simulink model "my_dom_trans_2013"  (R2013a)
settings: Solver=ode45  SolverMode=SingleTasking  StartTime=0.0  StopTime=10000  RelTol=1e-3
undefined symbols (not defined in the file): d_T_z, d_T_zew, L1, L2, M1, M2, steptime, T_p0, T_wew0
settings Model: CovMetricSettings=dwe  CovHtmlReporting=off  covSaveCumulativeToWorkspaceVar=off  CovSaveSingleToWorkspaceVar=off  CovExternalEMLEnable=on  Creator=johnb  LastModifiedBy=johnb
settings DataIOCC: LimitDataPoints=off  SaveFormat=StructureWithTime
settings DebuggingCC: UnderspecifiedInitializationDetection=Simplified  MergeDetectMultiDrivingBlocksExec=error  SolverPrmCheckMsg=none  FrameProcessingCompatibilityMsg=error  StateNameClashWarn=none  SFUnexpectedBacktrackingDiag=error  SFNoUnconditionalDefaultTransitionDiag=error
settings HardwareCC: ProdBitPerPointer=64  ProdLargestAtomicFloat=Float  ProdIntDivRoundTo=Zero  ProdEndianess=LittleEndian  ProdHWDeviceType=Specified
settings ModelReferenceCC: PropagateSignalLabelsOutOfModel=on
settings GRTTargetCC: CodeReplacementLibrary=C99 (ISO)  GeneratePreprocessorConditionals=Use local settings

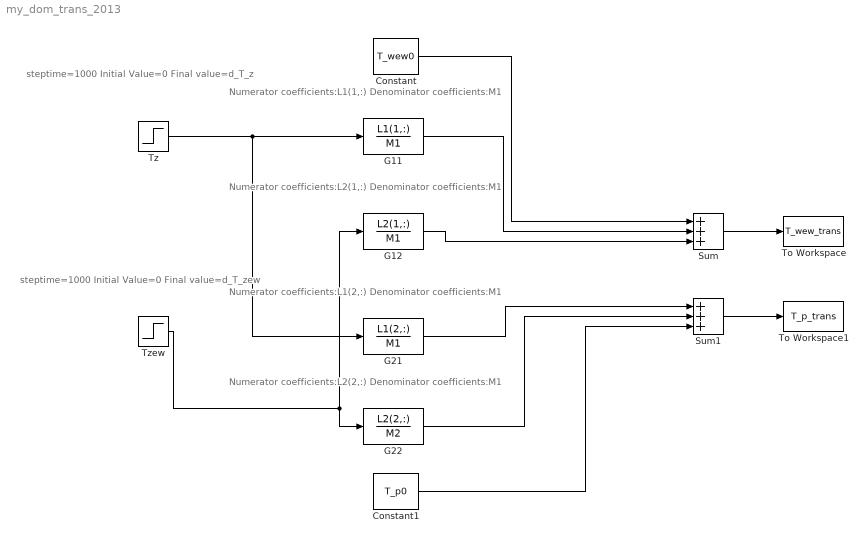
== system my_dom_trans_2013 ==
  note: Numerator coefficients:L1(1,:)
      | Denominator coefficients:M1
  note: steptime=1000
      | Initial Value=0
      | Final value=d_T_z
  note: steptime=1000
      | Initial Value=0
      | Final value=d_T_zew
  note: Numerator coefficients:L2(1,:)
      | Denominator coefficients:M1
  note: Numerator coefficients:L1(2,:)
      | Denominator coefficients:M1
  note: Numerator coefficients:L2(2,:)
      | Denominator coefficients:M1
  Constant : Constant  Value=T_wew0
  Constant1 : Constant  Value=T_p0
  G11 : TransferFcn  Numerator=L1(1,:)  Denominator=M1
  G12 : TransferFcn  Numerator=L2(1,:)  Denominator=M1
  G21 : TransferFcn  Numerator=L1(2,:)  Denominator=M1
  G22 : TransferFcn  Numerator=L2(2,:)  Denominator=M2
  Sum : Sum  Inputs=3
  Sum1 : Sum  Inputs=3
  To Workspace : ToWorkspace  VariableName=T_wew_trans  SaveFormat=Timeseries  SampleTime=-1
  To Workspace1 : ToWorkspace  VariableName=T_p_trans  SaveFormat=Timeseries  SampleTime=-1
  Tz : Step  Time=steptime  After=d_T_z  SampleTime=0
  "Tzew " : Step  Time=steptime  After=d_T_zew  SampleTime=0
  wires:
  Sum/1 -> To Workspace/1
  Sum1/1 -> To Workspace1/1
  Tz/1 -> G11/1, G21/1
  "Tzew "/1 -> G12/1, G22/1
  Constant/1 -> Sum/1
  G11/1 -> Sum/2
  G12/1 -> Sum/3
  G21/1 -> Sum1/1
  G22/1 -> Sum1/2
  Constant1/1 -> Sum1/3
